simulink model "Exo_Origianl"  (R2023b)
settings: Solver=ode5  StartTime=0.0  StopTime=inf  FixedStep=dt  RelTol=1e-3  EnableMultiTasking=on
values from neighbouring files (symbols this model uses):
  A_0_a = 4.011    [Operator.m]
  A_0_h = 40.69    [Operator.m]
  A_0_k = 25.7    [Operator.m]
  A_1_a = 5.292    [Operator.m]
  A_1_h = 23.22    [Operator.m]
  A_1_k = -3.827    [Operator.m]
  A_2_a = -8.582    [Operator.m]
  A_2_h = -4.487    [Operator.m]
  A_2_k = -8.543    [Operator.m]
  A_3_a = -0.4755    [Operator.m]
  A_3_h = 0.3995    [Operator.m]
  A_3_k = 1.913    [Operator.m]
  A_4_a = 1.688    [Operator.m]
  A_4_k = 1.087    [Operator.m]
  A_5_a = -0.03504    [Operator.m]
  A_5_k = 2.054    [Operator.m]
  A_6_a = 1.298    [Operator.m]
  A_6_k = -0.3061    [Operator.m]
  amplitude = 0.8    [Operator.m]
  ankleStrategyInterval = 1.5    [Operator.m]
  B_1_a = 3.613    [Operator.m]
  B_1_h = -8.65    [Operator.m]
  B_1_k = -19.28    [Operator.m]
  B_2_a = -5.954    [Operator.m]
  B_2_h = 3.338    [Operator.m]
  B_2_k = 17.93    [Operator.m]
  B_3_a = 5.918    [Operator.m]
  B_3_h = 1.389    [Operator.m]
  B_3_k = 3.772    [Operator.m]
  B_4_a = -2.118    [Operator.m]
  B_4_k = 1.504    [Operator.m]
  B_5_a = 1.023    [Operator.m]
  B_5_k = 0.5838    [Operator.m]
  B_6_a = -0.7245    [Operator.m]
  B_6_k = -0.8958    [Operator.m]
  DCM_filter = 1 - dt/(dt+RC)    (= 0.926612305411)    [Operator.m]
  dt = 0.01    [Operator.m]
  frequency = 1.2    [Operator.m]
  gamma = fzero(eqn, 0.1)    [Operator.m]
  hipOffset = -17    [Operator.m]
  K_high = 0.5    [Operator.m]
  K_low = 0.5    [Operator.m]
  KD = 0.39    [Operator.m]
  Kp = 10    [Operator.m]
  l3 = userHeight*0.232    (= 15.776)    [Operator.m]
  l4 = userHeight*0.247    (= 16.796)    [Operator.m]
  l_c2 = ((0.29*34.66+0.63*6.07)/(6.07+34.66))/(0.52+0.19)*l2    (= 15.0425832454)    [Operator.m]
  l_c3 = 0.17/0.40*l3    (= 6.7048)    [Operator.m]
  l_c4 = ((0.19*3.52+0.43*1.05)/(3.52+1.05))/0.43*l4    (= 9.57536959951)    [Operator.m]
  l_foot = 11.25    [Operator.m]
  m2 = m2 + 2.2048*7.591    (= 119.8566368)    [Operator.m]
  m3 = m3 + 2.2048*1.715    (= 19.781232)    [Operator.m]
  m4 = userWeight*(0.0459+0.0169)    (= 10.048)    [Operator.m]
  m_Exo = 2.2048*1.647    (= 3.6313056)    [Operator.m]
  m_f = userWeight*0.0169    (= 2.704)    [Operator.m]
  maxTorque = 35    [Operator.m]
  P_t_ZMP_gain_Ankle = 0    [Operator.m]
  P_t_ZMP_gain_Hip = 0    [Operator.m]
  Phase_Left = 2+pi    (= 5.14159265359)    [Operator.m]
  Phase_Right = 2    [Operator.m]
  ramp = 2    [Operator.m]
  Strategy_filter = DCM_filter    (= 0.926612305411)    [Operator.m]
  strategySaturation = 10    [Operator.m]
  userHeight = 68    [Operator.m]
  userWeight = 160    [Operator.m]
undefined symbols (not defined in the file or in its folder): CAN_Device, DCMErrorPenalty, PEAK, Phase_Left_Knee_0, System, totalPowerPenalty
libraries: sldrtlib x35, simulink x16, rllib x1
(part 3 of 4)

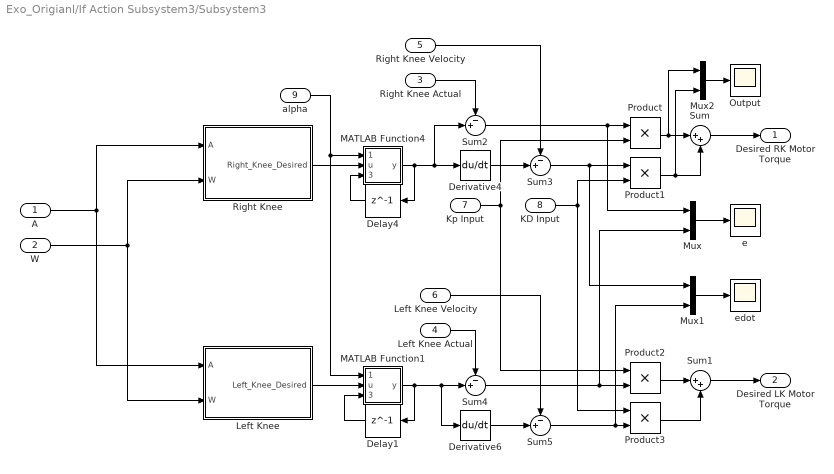
== system Exo_Origianl/If Action Subsystem3/Subsystem3 ==
  A : Inport
  W : Inport  Port=2
  Right Knee Actual : Inport  Port=3
  Left Knee Actual : Inport  Port=4
  Right Knee Velocity : Inport  Port=5
  Left Knee Velocity : Inport  Port=6
  Kp Input : Inport  Port=7
  KD Input : Inport  Port=8
  alpha : Inport  Port=9
  Delay1 : Delay  DelayLength=1
  Delay4 : Delay  DelayLength=1
  Derivative4 : Derivative
  Derivative6 : Derivative
  Left Knee : Subsystem
  MATLAB Function1 : MATLAB Function  TreatAsAtomicUnit=on
  MATLAB Function4 : MATLAB Function  TreatAsAtomicUnit=on
  Mux : Mux  Inputs=2
  Mux1 : Mux  Inputs=2
  Mux2 : Mux  Inputs=2
  Output : Scope
  Product{,1..3} (4 alike) : Product
  Right Knee : Subsystem
  Sum : Sum  Inputs=|++
  Sum1 : Sum  Inputs=|++
  Sum{2..5} (4 alike) : Sum  Inputs=-+|
  e : Scope
  edot : Scope
  Desired RK Motor Torque : Outport
  Desired LK Motor Torque : Outport  Port=2
  wires:
  KD Input/1 -> Product3/1, Product1/2
  Kp Input/1 -> Product2/1, Product/2
  Product3/1 -> Sum1/2
  W/1 -> Left Knee/2(W), Right Knee/2(W)
  Product1/1 -> Mux2/2, Sum/2
  Sum4/1 -> Mux/2, Product2/2
  Sum/1 -> Desired RK Motor Torque/1
  Sum2/1 -> Mux/1, Product/1
  Product/1 -> Mux2/1, Sum/1
  Product2/1 -> Sum1/1
  Sum3/1 -> Mux1/1, Product1/1
  Sum1/1 -> Desired LK Motor Torque/1
  Sum5/1 -> Mux1/2, Product3/2
  Mux/1 -> e/1
  Mux1/1 -> edot/1
  Right Knee Actual/1 -> Sum2/1
  Derivative4/1 -> Sum3/2
  Right Knee Velocity/1 -> Sum3/1
  Left Knee Actual/1 -> Sum4/1
  Derivative6/1 -> Sum5/2
  Left Knee Velocity/1 -> Sum5/1
  Mux2/1 -> Output/1
  MATLAB Function4/1(y) -> Sum2/2, Derivative4/1, Delay4/1
  MATLAB Function1/1(y) -> Derivative6/1, Sum4/2, Delay1/1
  A/1 -> Right Knee/1(A), Left Knee/1(A)
  Right Knee/1(Right_Knee_Desired) -> MATLAB Function4/2(u)
  Delay4/1 -> MATLAB Function4/3(y_delay)
  alpha/1 -> MATLAB Function4/1(alpha), MATLAB Function1/1(alpha)
  Left Knee/1(Left_Knee_Desired) -> MATLAB Function1/2(u)
  Delay1/1 -> MATLAB Function1/3(y_delay)

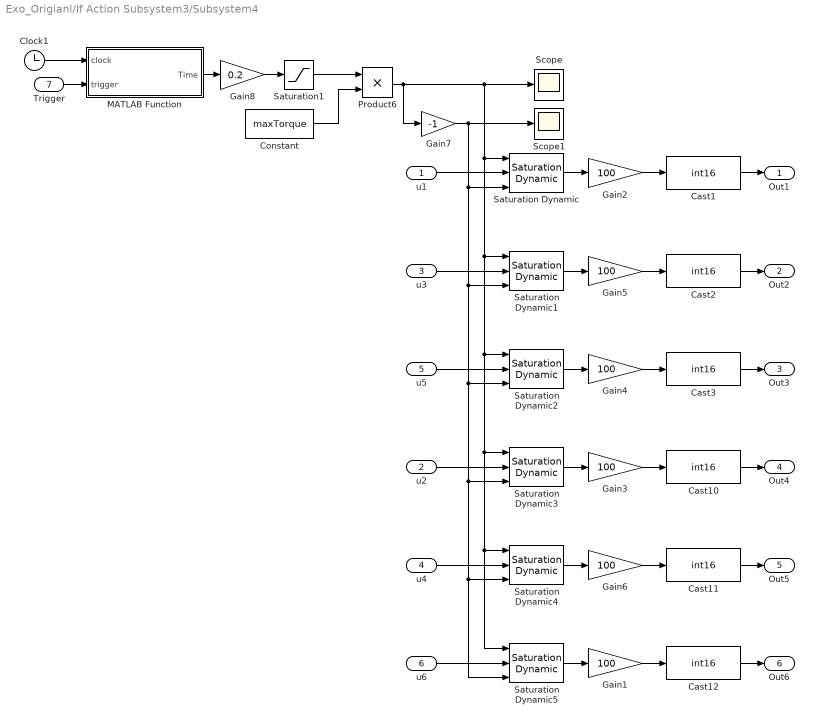
== system Exo_Origianl/If Action Subsystem3/Subsystem4 ==
  u1 : Inport
  u2 : Inport  Port=2
  u3 : Inport  Port=3
  u4 : Inport  Port=4
  u5 : Inport  Port=5
  u6 : Inport  Port=6
  Trigger : Inport  Port=7
  Cast{1..3,10..12} (6 alike) : DataTypeConversion  OutDataTypeStr=int16  SaturateOnIntegerOverflow=off  RndMeth=Floor
  Clock1 : Clock
  Constant : Constant  Value=maxTorque
  Gain{1..6} (6 alike) : Gain  Gain=100
  Gain7 : Gain  Gain=-1
  Gain8 : Gain  Gain=0.2
  MATLAB Function : MATLAB Function  TreatAsAtomicUnit=on
  Product6 : Product
  Saturation Dynamic{,1..5} (6 alike) : simulink/Discontinuities/Saturation Dynamic  OutMin=[]  OutMax=[]  OutDataTypeStr=Inherit: Same as second input  OutDataType=fixdt(1, 16)  OutScaling=2^-10  DoSatur=off
  Saturation1 : Saturate  UpperLimit=1  LowerLimit=0
  Scope : Scope
  Scope1 : Scope
  Out1 : Outport
  Out2 : Outport  Port=2
  Out3 : Outport  Port=3
  Out4 : Outport  Port=4
  Out5 : Outport  Port=5
  Out6 : Outport  Port=6
  wires:
  Gain2/1 -> Cast1/1
  Cast10/1 -> Out4/1
  Cast11/1 -> Out5/1
  Gain4/1 -> Cast3/1
  Gain3/1 -> Cast10/1
  Cast3/1 -> Out3/1
  Cast12/1 -> Out6/1
  Gain5/1 -> Cast2/1
  Gain6/1 -> Cast11/1
  Cast1/1 -> Out1/1
  Gain1/1 -> Cast12/1
  Cast2/1 -> Out2/1
  Saturation Dynamic/1 -> Gain2/1
  Saturation Dynamic1/1 -> Gain5/1
  Saturation Dynamic2/1 -> Gain4/1
  Saturation Dynamic3/1 -> Gain3/1
  Saturation Dynamic4/1 -> Gain6/1
  Saturation Dynamic5/1 -> Gain1/1
  Product6/1 -> Scope/1, Saturation Dynamic5/1, Saturation Dynamic4/1, Saturation Dynamic3/1, Saturation Dynamic2/1, Saturation Dynamic1/1, Saturation Dynamic/1, Gain7/1
  Gain7/1 -> Saturation Dynamic5/3, Saturation Dynamic4/3, Saturation Dynamic3/3, Saturation Dynamic2/3, Saturation Dynamic1/3, Saturation Dynamic/3, Scope1/1
  Gain8/1 -> Saturation1/1
  Clock1/1 -> MATLAB Function/1(clock)
  u1/1 -> Saturation Dynamic/2
  u3/1 -> Saturation Dynamic1/2
  u5/1 -> Saturation Dynamic2/2
  u2/1 -> Saturation Dynamic3/2
  u4/1 -> Saturation Dynamic4/2
  u6/1 -> Saturation Dynamic5/2
  Constant/1 -> Product6/2
  Saturation1/1 -> Product6/1
  MATLAB Function/1(Time) -> Gain8/1
  Trigger/1 -> MATLAB Function/2(trigger)

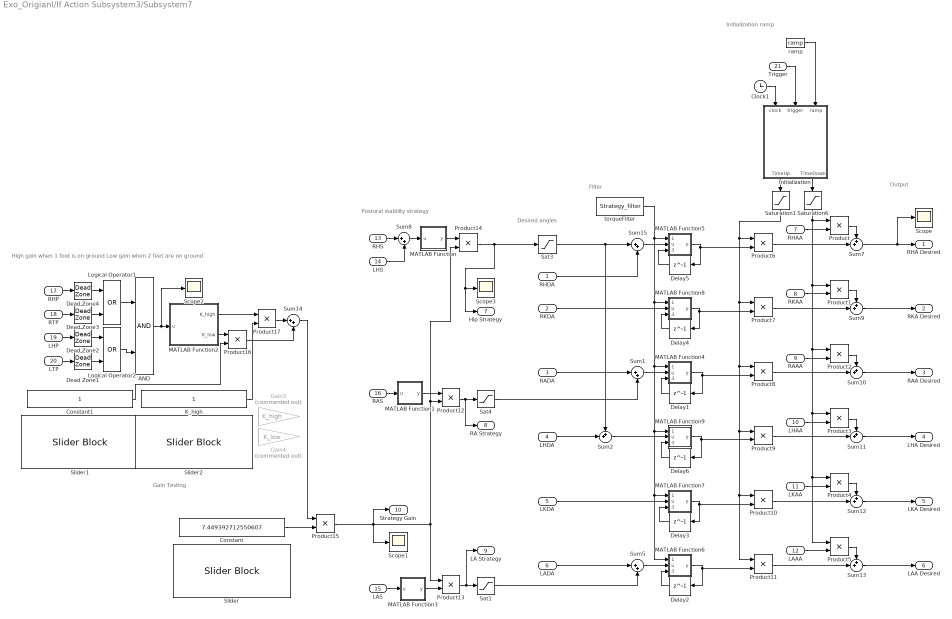
== system Exo_Origianl/If Action Subsystem3/Subsystem7 ==
  note: Gain Testing
  note: Output
  note: Initialization ramp
  note: Filter
  note: Desired angles
  note: Postural stability strategy
  note: High gain when 1 foot is on ground
      | Low gain when 2 feet are on ground
  RHDA : Inport
  RKDA : Inport  Port=2
  RADA : Inport  Port=3
  LHDA : Inport  Port=4
  LKDA : Inport  Port=5
  LADA : Inport  Port=6
  RHAA : Inport  Port=7
  RKAA : Inport  Port=8
  RAAA : Inport  Port=9
  LHAA : Inport  Port=10
  LKAA : Inport  Port=11
  LAAA : Inport  Port=12
  RHS : Inport  Port=13
  LHS : Inport  Port=14
  LAS : Inport  Port=15
  RAS : Inport  Port=16
  RHP : Inport  Port=17
  RTP : Inport  Port=18
  LHP : Inport  Port=19
  LTP : Inport  Port=20
  Trigger : Inport  Port=21
  AND : Logic  IconShape=distinctive  AllPortsSameDT=off  OutDataTypeStr=boolean
  Clock1 : Clock
  Constant : Constant  Value=7.449392712550607
  Constant1 : Constant
  Dead Zone{1..4} (4 alike) : DeadZone  LowerValue=0  UpperValue=pressureDeadZone
  Delay{1..6} (6 alike) : Delay  DelayLength=1
  Gain3 : Gain  Commented=on  Gain=K_high
  Gain4 : Gain  Commented=on  Gain=K_low
  Initialization : MATLAB Function  TreatAsAtomicUnit=on
  K_high : Constant
  Logical Operator1 : Logic  Operator=OR  AllPortsSameDT=off  OutDataTypeStr=boolean
  Logical Operator2 : Logic  Operator=OR  AllPortsSameDT=off  OutDataTypeStr=boolean
  MATLAB Function : MATLAB Function  TreatAsAtomicUnit=on
  MATLAB Function1 : MATLAB Function  TreatAsAtomicUnit=on
  MATLAB Function2 : MATLAB Function  TreatAsAtomicUnit=on
  MATLAB Function3 : MATLAB Function  TreatAsAtomicUnit=on
  MATLAB Function4 : MATLAB Function  TreatAsAtomicUnit=on
  MATLAB Function5 : MATLAB Function  TreatAsAtomicUnit=on
  MATLAB Function6 : MATLAB Function  TreatAsAtomicUnit=on
  MATLAB Function7 : MATLAB Function  TreatAsAtomicUnit=on
  MATLAB Function8 : MATLAB Function  TreatAsAtomicUnit=on
  MATLAB Function9 : MATLAB Function  TreatAsAtomicUnit=on
  Product{,1..17} (18 alike) : Product
  Sat1 : Saturate  UpperLimit=strategySaturation  LowerLimit=-strategySaturation
  Sat3 : Saturate  UpperLimit=strategySaturation  LowerLimit=-strategySaturation
  Sat4 : Saturate  UpperLimit=strategySaturation  LowerLimit=-strategySaturation
  Saturation1 : Saturate  UpperLimit=1  LowerLimit=0
  Saturation6 : Saturate  UpperLimit=1  LowerLimit=0
  Scope{,1..3} (4 alike) : Scope
  Slider : SliderBlock  ScaleMax=10
  Slider1 : SliderBlock  ScaleMin=0.5  ScaleMax=1
  Slider2 : SliderBlock  ScaleMin=1  ScaleMax=3
  Sum{1,5,8,14..15} (5 alike) : Sum  Inputs=|++
  Sum{2,7,9..13} (7 alike) : Sum  Inputs=++|
  ramp : Constant  Value=ramp
  torqueFilter : Constant  Value=Strategy_filter
  RHA Desired : Outport
  RKA Desired : Outport  Port=2
  RAA Desired : Outport  Port=3
  LHA Desired : Outport  Port=4
  LKA Desired : Outport  Port=5
  LAA Desired : Outport  Port=6
  Hip Strategy : Outport  Port=7
  RA Strategy : Outport  Port=8
  LA Strategy : Outport  Port=9
  Strategy Gain : Outport  Port=10
  wires:
  RHS/1 -> Sum8/1
  LADA/1 -> Sum5/1
  LHDA/1 -> Sum2/2
  Sum2/1 -> MATLAB Function9/2(u)
  Sum13/1 -> LAA Desired/1
  Sum8/1 -> MATLAB Function/1(u)
  MATLAB Function6/1(y) -> Product11/2, Delay2/1
  RAS/1 -> MATLAB Function1/1(u)
  MATLAB Function4/1(y) -> Product8/2, Delay1/1
  MATLAB Function1/1(y) -> Product12/1
  Sum11/1 -> LHA Desired/1
  Sum7/1 -> RHA Desired/1, Scope/1
  Sum9/1 -> RKA Desired/1
  Sum10/1 -> RAA Desired/1
  Sum12/1 -> LKA Desired/1
  RADA/1 -> Sum1/1
  LHS/1 -> Sum8/2
  LAS/1 -> MATLAB Function3/1(u)
  RKDA/1 -> MATLAB Function8/2(u)
  LKDA/1 -> MATLAB Function7/2(u)
  Trigger/1 -> Initialization/2(trigger)
  Clock1/1 -> Initialization/1(clock)
  RHAA/1 -> Product/2
  RKAA/1 -> Product1/2
  RAAA/1 -> Product2/2
  LHAA/1 -> Product3/2
  LKAA/1 -> Product4/2
  LAAA/1 -> Product5/2
  Initialization/2(TimeDown) -> Saturation6/1
  Delay5/1 -> MATLAB Function5/3(y_delay)
  torqueFilter/1 -> MATLAB Function5/1(alpha), MATLAB Function9/1(alpha), MATLAB Function7/1(alpha), MATLAB Function6/1(alpha), MATLAB Function4/1(alpha), MATLAB Function8/1(alpha)
  Delay1/1 -> MATLAB Function4/3(y_delay)
  Delay2/1 -> MATLAB Function6/3(y_delay)
  MATLAB Function5/1(y) -> Product6/2, Delay5/1
  RHP/1 -> Dead Zone4/1
  RTP/1 -> Dead Zone3/1
  LHP/1 -> Dead Zone2/1
  LTP/1 -> Dead Zone1/1
  Logical Operator1/1 -> AND/1
  Product12/1 -> Sat4/1, RA Strategy/1
  Product13/1 -> LA Strategy/1, Sat1/1
  Logical Operator2/1 -> AND/2
  MATLAB Function3/1(y) -> Product13/2
  Saturation6/1 -> Product5/1, Product4/1, Product3/1, Product2/1, Product1/1, Product/1
  Product/1 -> Sum7/1
  Product1/1 -> Sum9/1
  Product2/1 -> Sum10/1
  Product3/1 -> Sum11/1
  Product4/1 -> Sum12/1
  Product5/1 -> Sum13/1
  Dead Zone4/1 -> Logical Operator1/1
  Dead Zone3/1 -> Logical Operator1/2
  Dead Zone2/1 -> Logical Operator2/1
  Dead Zone1/1 -> Logical Operator2/2
  MATLAB Function2/1(K_high) -> Product17/1
  MATLAB Function2/2(K_low) -> Product16/1
  Product16/1 -> Sum14/2
  Product17/1 -> Sum14/1
  ramp/1 -> Initialization/3(ramp)
  AND/1 -> Scope2/1, MATLAB Function2/1(u)
  Sum15/1 -> MATLAB Function5/2(u)
  RHDA/1 -> Sum15/2
  Sum5/1 -> MATLAB Function6/2(u)
  Delay3/1 -> MATLAB Function7/3(y_delay)
  MATLAB Function7/1(y) -> Product10/2, Delay3/1
  Sum1/1 -> MATLAB Function4/2(u)
  Delay4/1 -> MATLAB Function8/3(y_delay)
  MATLAB Function8/1(y) -> Product7/2, Delay4/1
  Delay6/1 -> MATLAB Function9/3(y_delay)
  MATLAB Function9/1(y) -> Product9/2, Delay6/1
  Initialization/1(TimeUp) -> Saturation1/1
  Product6/1 -> Sum7/2
  Saturation1/1 -> Product10/1, Product11/1, Product9/1, Product8/1, Product7/1, Product6/1
  Product7/1 -> Sum9/2
  Product8/1 -> Sum10/2
  Product9/1 -> Sum11/2
  Product10/1 -> Sum12/2
  Product11/1 -> Sum13/2
  Product14/1 -> Scope3/1, Hip Strategy/1, Sat3/1
  MATLAB Function/1(y) -> Product14/1
  Product15/1 -> Scope1/1, Strategy Gain/1, Product14/2, Product12/2, Product13/1
  Sat3/1 -> Sum2/1, Sum15/1
  Sat4/1 -> Sum1/2
  Sat1/1 -> Sum5/2
  Sum14/1 -> Product15/1
  Constant/1 -> Product15/2
  Constant1/1 -> Product16/2
  K_high/1 -> Product17/2

== system Exo_Origianl/Read Angular Possition/If Action Subsystem ==
  Action Port : ActionPort  ActionPortLabel=if(u1 == 1)
  Data Type Conversion{6..11} (6 alike) : DataTypeConversion  OutDataTypeStr=double  SaturateOnIntegerOverflow=off  RndMeth=Floor
  Packet Input1 : sldrtlib/Packet Input  SampleTime=-1  MaxMissedTicks=10  ShowMissedTicks=off  YieldWhenWaiting=off  DrvName=PEAK-System/CAN_Device  DrvAddress=81  DrvOptions=[0 0 0 0 1000 0 0 1 5 2 1 3 1]  PacketSize=6  DataTypes={'int8','int8','int8','int8','int8','int8'}  ShowReady=off  ShowError=off  PacketID=2048e0 + (110)  ByteOrder=1  ShowTimestamp=off
      settings: AttributesFormatString=PEAK-System\nCAN Device [81]
  Out7 : Outport
  Out8 : Outport  Port=2
  Out9 : Outport  Port=3
  Out10 : Outport  Port=4
  Out11 : Outport  Port=5
  Out12 : Outport  Port=6
  wires:
  Data Type Conversion10/1 -> Out11/1
  Packet Input1/6 -> Data Type Conversion11/1
  Data Type Conversion11/1 -> Out12/1
  Packet Input1/5 -> Data Type Conversion10/1
  Data Type Conversion7/1 -> Out8/1
  Packet Input1/4 -> Data Type Conversion9/1
  Data Type Conversion6/1 -> Out7/1
  Packet Input1/2 -> Data Type Conversion7/1
  Data Type Conversion8/1 -> Out9/1
  Packet Input1/1 -> Data Type Conversion6/1
  Data Type Conversion9/1 -> Out10/1
  Packet Input1/3 -> Data Type Conversion8/1

== system Exo_Origianl/Read Angular Possition/If Action Subsystem1 ==
  Action Port : ActionPort  ActionPortLabel=else
  Data Type Conversion{6..11} (6 alike) : DataTypeConversion  OutDataTypeStr=double  SaturateOnIntegerOverflow=off  RndMeth=Floor
  Multiply{,1..5} (6 alike) : Gain  Gain=0.1
  Packet Input1 : sldrtlib/Packet Input  SampleTime=-1  MaxMissedTicks=10000  ShowMissedTicks=off  YieldWhenWaiting=off  DrvName=PEAK-System/CAN_Device  DrvAddress=81  DrvOptions=[0 0 0 0 1000 0 0 1 5 2 1 3 1]  PacketSize=6  DataTypes={'int16','int16','int16'}  ShowReady=off  ShowError=off  PacketID=2048e0 + (50)  ByteOrder=1  ShowTimestamp=off
      settings: AttributesFormatString=PEAK-System\nCAN Device [81]
  Packet Input2 : sldrtlib/Packet Input  SampleTime=-1  MaxMissedTicks=1000  ShowMissedTicks=off  YieldWhenWaiting=off  DrvName=PEAK-System/CAN_Device  DrvAddress=81  DrvOptions=[0 0 0 0 1000 0 0 1 5 2 1 3 1]  PacketSize=6  DataTypes={'int16','int16','int16'}  ShowReady=off  ShowError=off  PacketID=2048e0 + (51)  ByteOrder=1  ShowTimestamp=off
      settings: AttributesFormatString=PEAK-System\nCAN Device [81]
  Out7 : Outport
  Out8 : Outport  Port=2
  Out9 : Outport  Port=3
  Out10 : Outport  Port=4
  Out11 : Outport  Port=5
  Out12 : Outport  Port=6
  wires:
  Packet Input2/1 -> Data Type Conversion9/1
  Packet Input1/3 -> Data Type Conversion8/1
  Packet Input1/2 -> Data Type Conversion7/1
  Packet Input2/3 -> Data Type Conversion11/1
  Packet Input2/2 -> Data Type Conversion10/1
  Packet Input1/1 -> Data Type Conversion6/1
  Data Type Conversion6/1 -> Multiply/1
  Multiply/1 -> Out7/1
  Data Type Conversion7/1 -> Multiply1/1
  Multiply1/1 -> Out8/1
  Data Type Conversion8/1 -> Multiply2/1
  Multiply2/1 -> Out9/1
  Data Type Conversion9/1 -> Multiply3/1
  Multiply3/1 -> Out10/1
  Data Type Conversion10/1 -> Multiply4/1
  Multiply4/1 -> Out11/1
  Data Type Conversion11/1 -> Multiply5/1
  Multiply5/1 -> Out12/1

== system Exo_Origianl/Read Angular Velocity/If Action Subsystem1 ==
  Action Port : ActionPort  ActionPortLabel=else
  Data Type Conversion{6..11} (6 alike) : DataTypeConversion  OutDataTypeStr=double  SaturateOnIntegerOverflow=off  RndMeth=Floor
  Multiply{,1..5} (6 alike) : Gain  Gain=0.1
  Packet Input1 : sldrtlib/Packet Input  SampleTime=-1  MaxMissedTicks=10000  ShowMissedTicks=off  YieldWhenWaiting=off  DrvName=PEAK-System/CAN_Device  DrvAddress=81  DrvOptions=[0 0 0 0 1000 0 0 1 5 2 1 3 1]  PacketSize=6  DataTypes={'int16','int16','int16'}  ShowReady=off  ShowError=off  PacketID=2048e0 + (52)  ByteOrder=1  ShowTimestamp=off
      settings: AttributesFormatString=PEAK-System\nCAN Device [81]
  Packet Input2 : sldrtlib/Packet Input  SampleTime=-1  MaxMissedTicks=1000  ShowMissedTicks=off  YieldWhenWaiting=off  DrvName=PEAK-System/CAN_Device  DrvAddress=81  DrvOptions=[0 0 0 0 1000 0 0 1 5 2 1 3 1]  PacketSize=6  DataTypes={'int16','int16','int16'}  ShowReady=off  ShowError=off  PacketID=2048e0 + (53)  ByteOrder=1  ShowTimestamp=off
      settings: AttributesFormatString=PEAK-System\nCAN Device [81]
  Out7 : Outport
  Out8 : Outport  Port=2
  Out9 : Outport  Port=3
  Out10 : Outport  Port=4
  Out11 : Outport  Port=5
  Out12 : Outport  Port=6
  wires:
  Packet Input2/1 -> Data Type Conversion9/1
  Packet Input1/3 -> Data Type Conversion8/1
  Packet Input1/2 -> Data Type Conversion7/1
  Packet Input2/3 -> Data Type Conversion11/1
  Packet Input2/2 -> Data Type Conversion10/1
  Packet Input1/1 -> Data Type Conversion6/1
  Data Type Conversion6/1 -> Multiply/1
  Multiply/1 -> Out7/1
  Data Type Conversion7/1 -> Multiply1/1
  Multiply1/1 -> Out8/1
  Data Type Conversion8/1 -> Multiply2/1
  Multiply2/1 -> Out9/1
  Data Type Conversion9/1 -> Multiply3/1
  Multiply3/1 -> Out10/1
  Data Type Conversion10/1 -> Multiply4/1
  Multiply4/1 -> Out11/1
  Data Type Conversion11/1 -> Multiply5/1
  Multiply5/1 -> Out12/1

== system Exo_Origianl/Read Interaction torque/If Action Subsystem ==
  Action Port : ActionPort  ActionPortLabel=if(u1 == 1)
  Data Type Conversion{6..11} (6 alike) : DataTypeConversion  OutDataTypeStr=double  SaturateOnIntegerOverflow=off  RndMeth=Floor
  Packet Input1 : sldrtlib/Packet Input  SampleTime=-1  MaxMissedTicks=10  ShowMissedTicks=off  YieldWhenWaiting=off  DrvName=PEAK-System/CAN_Device  DrvAddress=81  DrvOptions=[0 0 0 0 1000 0 0 1 5 2 1 3 1]  PacketSize=6  DataTypes={'int8','int8','int8','int8','int8','int8'}  ShowReady=off  ShowError=off  PacketID=2048e0 + (120)  ByteOrder=1  ShowTimestamp=off
      settings: AttributesFormatString=PEAK-System\nCAN Device [81]
  Out7 : Outport
  Out8 : Outport  Port=2
  Out9 : Outport  Port=3
  Out10 : Outport  Port=4
  Out11 : Outport  Port=5
  Out12 : Outport  Port=6
  wires:
  Data Type Conversion10/1 -> Out11/1
  Packet Input1/6 -> Data Type Conversion11/1
  Data Type Conversion11/1 -> Out12/1
  Packet Input1/5 -> Data Type Conversion10/1
  Data Type Conversion7/1 -> Out8/1
  Packet Input1/4 -> Data Type Conversion9/1
  Data Type Conversion6/1 -> Out7/1
  Packet Input1/2 -> Data Type Conversion7/1
  Data Type Conversion8/1 -> Out9/1
  Packet Input1/1 -> Data Type Conversion6/1
  Data Type Conversion9/1 -> Out10/1
  Packet Input1/3 -> Data Type Conversion8/1

== system Exo_Origianl/Read Interaction torque/If Action Subsystem1 ==
  Action Port : ActionPort  ActionPortLabel=else
  Data Type Conversion{6..11} (6 alike) : DataTypeConversion  OutDataTypeStr=double  SaturateOnIntegerOverflow=off  RndMeth=Floor
  Multiply{,1..5} (6 alike) : Gain  Gain=0.1
  Packet Input1 : sldrtlib/Packet Input  SampleTime=-1  MaxMissedTicks=10000  ShowMissedTicks=off  YieldWhenWaiting=off  DrvName=PEAK-System/CAN_Device  DrvAddress=81  DrvOptions=[0 0 0 0 1000 0 0 1 5 2 1 3 1]  PacketSize=6  DataTypes={'int16','int16','int16'}  ShowReady=off  ShowError=off  PacketID=2048e0 + (54)  ByteOrder=1  ShowTimestamp=off
      settings: AttributesFormatString=PEAK-System\nCAN Device [81]
  Packet Input2 : sldrtlib/Packet Input  SampleTime=-1  MaxMissedTicks=1000  ShowMissedTicks=off  YieldWhenWaiting=off  DrvName=PEAK-System/CAN_Device  DrvAddress=81  DrvOptions=[0 0 0 0 1000 0 0 1 5 2 1 3 1]  PacketSize=6  DataTypes={'int16','int16','int16'}  ShowReady=off  ShowError=off  PacketID=2048e0 + (55)  ByteOrder=1  ShowTimestamp=off
      settings: AttributesFormatString=PEAK-System\nCAN Device [81]
  Out7 : Outport
  Out8 : Outport  Port=2
  Out9 : Outport  Port=3
  Out10 : Outport  Port=4
  Out11 : Outport  Port=5
  Out12 : Outport  Port=6
  wires:
  Packet Input2/1 -> Data Type Conversion9/1
  Packet Input1/3 -> Data Type Conversion8/1
  Packet Input1/2 -> Data Type Conversion7/1
  Packet Input2/3 -> Data Type Conversion11/1
  Packet Input2/2 -> Data Type Conversion10/1
  Packet Input1/1 -> Data Type Conversion6/1
  Data Type Conversion6/1 -> Multiply/1
  Multiply/1 -> Out7/1
  Data Type Conversion7/1 -> Multiply1/1
  Multiply1/1 -> Out8/1
  Data Type Conversion8/1 -> Multiply2/1
  Multiply2/1 -> Out9/1
  Data Type Conversion9/1 -> Multiply3/1
  Multiply3/1 -> Out10/1
  Data Type Conversion10/1 -> Multiply4/1
  Multiply4/1 -> Out11/1
  Data Type Conversion11/1 -> Multiply5/1
  Multiply5/1 -> Out12/1

== system Exo_Origianl/Read Motor torque/If Action Subsystem ==
  Action Port : ActionPort  ActionPortLabel=if(u1 == 1)
  Data Type Conversion{6..11} (6 alike) : DataTypeConversion  OutDataTypeStr=double  SaturateOnIntegerOverflow=off  RndMeth=Floor
  Packet Input1 : sldrtlib/Packet Input  SampleTime=-1  MaxMissedTicks=10  ShowMissedTicks=off  YieldWhenWaiting=off  DrvName=PEAK-System/CAN_Device  DrvAddress=81  DrvOptions=[0 0 0 0 1000 0 0 1 5 2 1 3 1]  PacketSize=6  DataTypes={'int8','int8','int8','int8','int8','int8'}  ShowReady=off  ShowError=off  PacketID=2048e0 + (140)  ByteOrder=1  ShowTimestamp=off
      settings: AttributesFormatString=PEAK-System\nCAN Device [81]
  Out7 : Outport
  Out8 : Outport  Port=2
  Out9 : Outport  Port=3
  Out10 : Outport  Port=4
  Out11 : Outport  Port=5
  Out12 : Outport  Port=6
  wires:
  Data Type Conversion10/1 -> Out11/1
  Packet Input1/6 -> Data Type Conversion11/1
  Data Type Conversion11/1 -> Out12/1
  Packet Input1/5 -> Data Type Conversion10/1
  Data Type Conversion7/1 -> Out8/1
  Packet Input1/4 -> Data Type Conversion9/1
  Data Type Conversion6/1 -> Out7/1
  Packet Input1/2 -> Data Type Conversion7/1
  Data Type Conversion8/1 -> Out9/1
  Packet Input1/1 -> Data Type Conversion6/1
  Data Type Conversion9/1 -> Out10/1
  Packet Input1/3 -> Data Type Conversion8/1

== system Exo_Origianl/Read Motor torque/If Action Subsystem1 ==
  Action Port : ActionPort  ActionPortLabel=else
  Data Type Conversion{6..11} (6 alike) : DataTypeConversion  OutDataTypeStr=double  SaturateOnIntegerOverflow=off  RndMeth=Floor
  Multiply{,1..5} (6 alike) : Gain  Gain=0.1
  Packet Input1 : sldrtlib/Packet Input  SampleTime=-1  MaxMissedTicks=10000  ShowMissedTicks=off  YieldWhenWaiting=off  DrvName=PEAK-System/CAN_Device  DrvAddress=81  DrvOptions=[0 0 0 0 1000 0 0 1 5 2 1 3 1]  PacketSize=6  DataTypes={'int16','int16','int16'}  ShowReady=off  ShowError=off  PacketID=2048e0 + (56)  ByteOrder=1  ShowTimestamp=off
      settings: AttributesFormatString=PEAK-System\nCAN Device [81]
  Packet Input2 : sldrtlib/Packet Input  SampleTime=-1  MaxMissedTicks=1000  ShowMissedTicks=off  YieldWhenWaiting=off  DrvName=PEAK-System/CAN_Device  DrvAddress=81  DrvOptions=[0 0 0 0 1000 0 0 1 5 2 1 3 1]  PacketSize=6  DataTypes={'int16','int16','int16'}  ShowReady=off  ShowError=off  PacketID=2048e0 + (57)  ByteOrder=1  ShowTimestamp=off
      settings: AttributesFormatString=PEAK-System\nCAN Device [81]
  Out7 : Outport
  Out8 : Outport  Port=2
  Out9 : Outport  Port=3
  Out10 : Outport  Port=4
  Out11 : Outport  Port=5
  Out12 : Outport  Port=6
  wires:
  Packet Input2/1 -> Data Type Conversion9/1
  Packet Input1/3 -> Data Type Conversion8/1
  Packet Input1/2 -> Data Type Conversion7/1
  Packet Input2/3 -> Data Type Conversion11/1
  Packet Input2/2 -> Data Type Conversion10/1
  Packet Input1/1 -> Data Type Conversion6/1
  Data Type Conversion6/1 -> Multiply/1
  Multiply/1 -> Out7/1
  Data Type Conversion7/1 -> Multiply1/1
  Multiply1/1 -> Out8/1
  Data Type Conversion8/1 -> Multiply2/1
  Multiply2/1 -> Out9/1
  Data Type Conversion9/1 -> Multiply3/1
  Multiply3/1 -> Out10/1
  Data Type Conversion10/1 -> Multiply4/1
  Multiply4/1 -> Out11/1
  Data Type Conversion11/1 -> Multiply5/1
  Multiply5/1 -> Out12/1

== system Exo_Origianl/Subsystem13/Subsystem14 ==
  DCM Error : Inport
  Power : Inport  Port=2
  "                    " : Gain  Gain=-totalPowerPenalty
  "                    1" : Gain  Gain=-DCMErrorPenalty
  Bus Creator1 : BusCreator  Inputs=2
  Constant : Constant  Value=4
  Constant1 : Constant  Value=2
  Math Function : Math  Operator=pow
  Math Function2 : Math  Operator=pow
  Sum of Elements : Sum  Inputs=+
  Reward : Outport  VectorParamsAs1DForOutWhenUnconnected=off
  wires:
  Power/1 -> Math Function2/2
  Constant1/1 -> Math Function2/1
  Constant/1 -> Math Function/1
  DCM Error/1 -> Math Function/2
  Math Function2/1 -> "                    "/1
  Math Function/1 -> "                    1"/1
  Sum of Elements/1 -> Reward/1
  Bus Creator1/1 -> Sum of Elements/1
  "                    1"/1 -> Bus Creator1/1  "DCM Penalty"
  "                    "/1 -> Bus Creator1/2  "Power Penalty"

== system Exo_Origianl/Subsystem15/Subsystem14 ==
  Input : Inport
  Constant12 : Constant  Value=0
  Constant3 : Constant
  Display4 : Display
  If Action Subsystem4 : Subsystem  TreatAsAtomicUnit=on
  If Action Subsystem5 : Subsystem  TreatAsAtomicUnit=on
  If Action Subsystem6 : Subsystem  TreatAsAtomicUnit=on
  If Action Subsystem7 : Subsystem  TreatAsAtomicUnit=on
  If Action Subsystem8 : Subsystem  TreatAsAtomicUnit=on
  If3 : If  IfExpression=u1 == 0  ElseIfExpressions=u1 == 11, u1 == 12, u1 == 19
  Merge1 : Merge  Inputs=5
  Out1 : Outport
  wires:
  Constant12/1 -> If Action Subsystem8/1(In1)
  If Action Subsystem4/1(Out1) -> Merge1/1
  If3/3 -> If Action Subsystem6/Action
  If3/4 -> If Action Subsystem7/Action
  If Action Subsystem5/1(Out1) -> Merge1/2
  If Action Subsystem7/1(Out1) -> Merge1/4
  If3/5 -> If Action Subsystem8/Action
  If3/1 -> If Action Subsystem4/Action
  Input/1 -> If3/1
  Merge1/1 -> Out1/1, Display4/1
  If Action Subsystem8/1(Out1) -> Merge1/5
  If3/2 -> If Action Subsystem5/Action
  Constant3/1 -> If Action Subsystem7/1(In1), If Action Subsystem6/1(In1), If Action Subsystem5/1(In1), If Action Subsystem4/1(In1)
  If Action Subsystem6/1(Out1) -> Merge1/3

== system Exo_Origianl/Up and Down Assistance % Left/Subsystem ==
  In1 : Inport
  In2 : Inport  Port=2
  Add : Sum  OutMin=[0]  OutMax=[10]
  Add1 : Sum  OutMin=[0]  OutMax=[10]
  Add2 : Sum
  Cast To Double : DataTypeConversion  OutDataTypeStr=double  SaturateOnIntegerOverflow=off  RndMeth=Floor
  Constant : Constant  Value=10
  Constant1 : Constant  Value=40
  Delay : Delay  DelayLength=1
  Delay1 : Delay  DelayLength=1
  Detect Rise Positive : simulink/Logic and Bit Operations/Detect Rise Positive  vinit=0  OutDataTypeStr=uint8
  Detect Rise Positive1 : simulink/Logic and Bit Operations/Detect Rise Positive  vinit=0  OutDataTypeStr=uint8
  Display1 : Display
  Display2 : Display
  Gain : Gain  Gain=10
  If : If  IfExpression=(u1 > 0)
  If Action Subsystem : Subsystem  TreatAsAtomicUnit=on
  If Action Subsystem1 : Subsystem  TreatAsAtomicUnit=on
  If1 : If  IfExpression=(u1 < 9)
  Minus : Sum  Inputs=+-
  Minus1 : Sum  Inputs=+-  OutMin=[0]  OutMax=[10]
  Out1 : Outport
  Out2 : Outport  Port=2
  wires:
  Detect Rise Positive1/1 -> Minus1/2
  Detect Rise Positive/1 -> Add/2
  Minus1/1 -> Delay1/1
  Add/1 -> Delay/1
  Add1/1 -> Cast To Double/1
  Cast To Double/1 -> If/1, Minus/2, If1/1, Display2/1
  If Action Subsystem/1(Out1) -> Detect Rise Positive/1
  If1/1 -> If Action Subsystem/Action
  If Action Subsystem1/1(Out1) -> Detect Rise Positive1/1
  If/1 -> If Action Subsystem1/Action
  In1/1 -> If Action Subsystem/1(In1)
  In2/1 -> If Action Subsystem1/1(In1)
  Delay/1 -> Add1/1, Display1/1, Add/1
  Delay1/1 -> Minus1/1, Add1/2
  Gain/1 -> Out1/1
  Constant/1 -> Minus/1
  Minus/1 -> Add2/1, Gain/1
  Constant1/1 -> Add2/2
  Add2/1 -> Out2/1

== system Exo_Origianl/Up and Down Assistance % Right/Subsystem ==
  In1 : Inport
  In2 : Inport  Port=2
  Add : Sum  OutMin=[0]  OutMax=[10]
  Add1 : Sum  OutMin=[0]  OutMax=[10]
  Add2 : Sum
  Cast To Double : DataTypeConversion  OutDataTypeStr=double  SaturateOnIntegerOverflow=off  RndMeth=Floor
  Constant : Constant  Value=10
  Constant1 : Constant  Value=30
  Delay : Delay  DelayLength=1
  Delay1 : Delay  DelayLength=1
  Detect Rise Positive : simulink/Logic and Bit Operations/Detect Rise Positive  vinit=0  OutDataTypeStr=uint8
  Detect Rise Positive1 : simulink/Logic and Bit Operations/Detect Rise Positive  vinit=0  OutDataTypeStr=uint8
  Display1 : Display
  Display2 : Display
  Gain : Gain  Gain=10
  If : If  IfExpression=(u1 > 0)
  If Action Subsystem : Subsystem  TreatAsAtomicUnit=on
  If Action Subsystem1 : Subsystem  TreatAsAtomicUnit=on
  If1 : If  IfExpression=(u1 < 9)
  Minus : Sum  Inputs=+-
  Minus1 : Sum  Inputs=+-  OutMin=[0]  OutMax=[10]
  Out1 : Outport
  Out2 : Outport  Port=2
  wires:
  Detect Rise Positive1/1 -> Minus1/2
  Detect Rise Positive/1 -> Add/2
  Minus1/1 -> Delay1/1
  Add/1 -> Delay/1
  Add1/1 -> Cast To Double/1
  Cast To Double/1 -> If/1, Minus/2, If1/1, Display2/1
  If Action Subsystem/1(Out1) -> Detect Rise Positive/1
  If1/1 -> If Action Subsystem/Action
  If Action Subsystem1/1(Out1) -> Detect Rise Positive1/1
  If/1 -> If Action Subsystem1/Action
  In1/1 -> If Action Subsystem/1(In1)
  In2/1 -> If Action Subsystem1/1(In1)
  Delay/1 -> Add1/1, Display1/1, Add/1
  Delay1/1 -> Minus1/1, Add1/2
  Gain/1 -> Out1/1
  Constant/1 -> Minus/1
  Minus/1 -> Add2/1, Gain/1
  Add2/1 -> Out2/1
  Constant1/1 -> Add2/2

== system Exo_Origianl/Up and Down Speed/Subsystem ==
  In1 : Inport
  In2 : Inport  Port=2
  Add : Sum  OutMin=[0]  OutMax=[10]
  Add1 : Sum  OutMin=[0]  OutMax=[10]
  Cast To Double : DataTypeConversion  OutDataTypeStr=double  SaturateOnIntegerOverflow=off  RndMeth=Floor
  Delay : Delay  DelayLength=1
  Delay1 : Delay  DelayLength=1
  Detect Rise Positive : simulink/Logic and Bit Operations/Detect Rise Positive  vinit=0  OutDataTypeStr=uint8
  Detect Rise Positive1 : simulink/Logic and Bit Operations/Detect Rise Positive  vinit=0  OutDataTypeStr=uint8
  Display1 : Display
  Display2 : Display
  If : If  IfExpression=(u1 > 1)
  If Action Subsystem : Subsystem  TreatAsAtomicUnit=on
  If Action Subsystem1 : Subsystem  TreatAsAtomicUnit=on
  If1 : If  IfExpression=(u1 < 10)
  Increment Stored Integer : simulink/Additional Math & Discrete/Additional Math: Increment - Decrement/Increment Stored Integer
  Minus1 : Sum  Inputs=+-  OutMin=[0]  OutMax=[10]
  Out1 : Outport
  wires:
  Detect Rise Positive1/1 -> Minus1/2
  Detect Rise Positive/1 -> Add/2
  Minus1/1 -> Delay1/1
  Delay/1 -> Add1/1, Display1/1, Add/1
  Add/1 -> Delay/1
  Delay1/1 -> Add1/2, Minus1/1
  Add1/1 -> Increment Stored Integer/1
  Increment Stored Integer/1 -> Cast To Double/1
  Cast To Double/1 -> If/1, Out1/1, If1/1, Display2/1
  If Action Subsystem/1(Out1) -> Detect Rise Positive/1
  If1/1 -> If Action Subsystem/Action
  If Action Subsystem1/1(Out1) -> Detect Rise Positive1/1
  If/1 -> If Action Subsystem1/Action
  In1/1 -> If Action Subsystem/1(In1)
  In2/1 -> If Action Subsystem1/1(In1)

== system Exo_Origianl/If Action Subsystem3/Fourier Series/Left Ankle ==
  A : Inport
  W : Inport  Port=2
  Constant : Constant  Value=Phase_Left
  Integrator1 : Integrator  ExternalReset=rising  InitialConditionSource=external  InitialCondition=Phase_Left_Knee_0
  Mux1 : Mux  Inputs=2
  Scope1 : Scope
  ankle walk : Fcn  Expr=u(1)*(A_0_a + A_1_a*cos(u(2)) + B_1_a*sin(u(2)) + A_2_a*cos(2*u(2)) + B_2_a*sin(2*u(2)) + A_3_a*cos(3*u(2)) + B_3_a*sin(3*u(2)) + A_4_a*cos(4*u(2)) + B_4_a*sin(4*u(2)) + A_5_a*cos(5*u(2)) + B_5_a*sin(5*u(2)) + A_6_a*cos(6*u(2)) + B_6_a*sin(6*u(2)))
  Left_Ankle_Desired : Outport
  wires:
  W/1 -> Integrator1/2, Integrator1/1
  Mux1/1 -> ankle walk/1
  Constant/1 -> Integrator1/3
  A/1 -> Mux1/1
  ankle walk/1 -> Left_Ankle_Desired/1
  Integrator1/1 -> Mux1/2, Scope1/1

== system Exo_Origianl/If Action Subsystem3/Fourier Series/Left Hip ==
  A : Inport
  W : Inport  Port=2
  Offset : Inport  Port=3
  Constant1 : Constant  Value=Phase_Left
  Integrator4 : Integrator  ExternalReset=rising  InitialConditionSource=external  InitialCondition=Phase_Left_Knee_0
  Mux6 : Mux  Inputs=3
  Scope : Scope
  hip walk : Fcn  Expr=(u(1)*(A_0_h + A_1_h*cos(u(2)) + A_2_h*cos(2*u(2)) + A_3_h*cos(3*u(2)) + B_1_h*sin(u(2)) + B_2_h*sin(2*u(2)) + B_3_h*sin(3*u(2))))+u(3)
  Left_Hip_Desired : Outport
  wires:
  W/1 -> Integrator4/2, Integrator4/1
  Mux6/1 -> hip walk/1
  Constant1/1 -> Integrator4/3
  A/1 -> Mux6/1
  hip walk/1 -> Left_Hip_Desired/1
  Offset/1 -> Mux6/3
  Integrator4/1 -> Scope/1, Mux6/2

== system Exo_Origianl/If Action Subsystem3/Fourier Series/Left Knee ==
  A : Inport
  W : Inport  Port=2
  Constant1 : Constant  Value=Phase_Left
  Integrator1 : Integrator  ExternalReset=rising  InitialConditionSource=external  InitialCondition=Phase_Left_Knee_0
  Mux1 : Mux  Inputs=2
  Scope4 : Scope
  knee walk : Fcn  Expr=u(1)*(A_0_k + A_1_k*cos(u(2)) + B_1_k*sin(u(2)) + A_2_k*cos(2*u(2)) + B_2_k*sin(2*u(2)) + A_3_k*cos(3*u(2)) + B_3_k*sin(3*u(2)) + A_4_k*cos(4*u(2)) + B_4_k*sin(4*u(2)) + A_5_k*cos(5*u(2)) + B_5_k*sin(5*u(2)) + A_6_k*cos(6*u(2)) + B_6_k*sin(6*u(2)))
  Left_Knee_Desired : Outport
  wires:
  A/1 -> Mux1/1
  W/1 -> Integrator1/2, Integrator1/1
  Integrator1/1 -> Mux1/2, Scope4/1
  Constant1/1 -> Integrator1/3
  Mux1/1 -> knee walk/1
  knee walk/1 -> Left_Knee_Desired/1

== system Exo_Origianl/If Action Subsystem3/Fourier Series/Right Ankle ==
  A : Inport
  W : Inport  Port=2
  Constant : Constant  Value=Phase_Right
  Integrator1 : Integrator  ExternalReset=rising  InitialConditionSource=external  InitialCondition=Phase_Left_Knee_0
  Mux1 : Mux  Inputs=2
  Scope1 : Scope
  ankle walk : Fcn  Expr=u(1)*(A_0_a + A_1_a*cos(u(2)) + B_1_a*sin(u(2)) + A_2_a*cos(2*u(2)) + B_2_a*sin(2*u(2)) + A_3_a*cos(3*u(2)) + B_3_a*sin(3*u(2)) + A_4_a*cos(4*u(2)) + B_4_a*sin(4*u(2)) + A_5_a*cos(5*u(2)) + B_5_a*sin(5*u(2)) + A_6_a*cos(6*u(2)) + B_6_a*sin(6*u(2)))
  Right_Ankle_Desired : Outport
  wires:
  W/1 -> Integrator1/2, Integrator1/1
  Mux1/1 -> ankle walk/1
  Constant/1 -> Integrator1/3
  A/1 -> Mux1/1
  ankle walk/1 -> Right_Ankle_Desired/1
  Integrator1/1 -> Mux1/2, Scope1/1

== system Exo_Origianl/If Action Subsystem3/Fourier Series/Right Hip ==
  A : Inport
  W : Inport  Port=2
  Offset : Inport  Port=3
  Constant1 : Constant  Value=Phase_Right
  Integrator4 : Integrator  ExternalReset=rising  InitialConditionSource=external  InitialCondition=Phase_Left_Knee_0
  Mux6 : Mux  Inputs=3
  Scope : Scope
  hip walk : Fcn  Expr=(u(1)*(A_0_h + A_1_h*cos(u(2)) + A_2_h*cos(2*u(2)) + A_3_h*cos(3*u(2)) + B_1_h*sin(u(2)) + B_2_h*sin(2*u(2)) + B_3_h*sin(3*u(2))))+u(3)
  Right_Hip_Desired : Outport
  wires:
  W/1 -> Integrator4/2, Integrator4/1
  Mux6/1 -> hip walk/1
  Constant1/1 -> Integrator4/3
  A/1 -> Mux6/1
  hip walk/1 -> Right_Hip_Desired/1
  Offset/1 -> Mux6/3
  Integrator4/1 -> Scope/1, Mux6/2

== system Exo_Origianl/If Action Subsystem3/Fourier Series/Right Knee ==
  W : Inport
  A : Inport  Port=2
  Constant1 : Constant  Value=Phase_Right
  Integrator1 : Integrator  ExternalReset=rising  InitialConditionSource=external  InitialCondition=Phase_Left_Knee_0
  Mux1 : Mux  Inputs=2
  Scope4 : Scope
  knee walk : Fcn  Expr=u(1)*(A_0_k + A_1_k*cos(u(2)) + B_1_k*sin(u(2)) + A_2_k*cos(2*u(2)) + B_2_k*sin(2*u(2)) + A_3_k*cos(3*u(2)) + B_3_k*sin(3*u(2)) + A_4_k*cos(4*u(2)) + B_4_k*sin(4*u(2)) + A_5_k*cos(5*u(2)) + B_5_k*sin(5*u(2)) + A_6_k*cos(6*u(2)) + B_6_k*sin(6*u(2)))
  Right_Knee_Desired : Outport
  wires:
  A/1 -> Mux1/1
  W/1 -> Integrator1/2, Integrator1/1
  Constant1/1 -> Integrator1/3
  Mux1/1 -> knee walk/1
  knee walk/1 -> Right_Knee_Desired/1
  Integrator1/1 -> Mux1/2, Scope4/1

== system Exo_Origianl/If Action Subsystem3/Subsystem/Left Ankle ==
  A : Inport
  W : Inport  Port=2
  Constant : Constant  Value=Phase_Left
  Integrator1 : Integrator  ExternalReset=rising  InitialConditionSource=external  InitialCondition=Phase_Left_Knee_0
  Mux1 : Mux  Inputs=2
  Scope1 : Scope
  ankle walk : Fcn  Expr=u(1)*(A_0_a + A_1_a*cos(u(2)) + B_1_a*sin(u(2)) + A_2_a*cos(2*u(2)) + B_2_a*sin(2*u(2)) + A_3_a*cos(3*u(2)) + B_3_a*sin(3*u(2)) + A_4_a*cos(4*u(2)) + B_4_a*sin(4*u(2)) + A_5_a*cos(5*u(2)) + B_5_a*sin(5*u(2)) + A_6_a*cos(6*u(2)) + B_6_a*sin(6*u(2)))
  Left_Ankle_Desired : Outport
  wires:
  W/1 -> Integrator1/2, Integrator1/1
  Mux1/1 -> ankle walk/1
  Constant/1 -> Integrator1/3
  A/1 -> Mux1/1
  ankle walk/1 -> Left_Ankle_Desired/1
  Integrator1/1 -> Mux1/2, Scope1/1

== system Exo_Origianl/If Action Subsystem3/Subsystem/Right Ankle ==
  A : Inport
  W : Inport  Port=2
  Constant : Constant  Value=Phase_Right
  Integrator1 : Integrator  ExternalReset=rising  InitialConditionSource=external  InitialCondition=Phase_Left_Knee_0
  Mux1 : Mux  Inputs=2
  Scope1 : Scope
  ankle walk : Fcn  Expr=u(1)*(A_0_a + A_1_a*cos(u(2)) + B_1_a*sin(u(2)) + A_2_a*cos(2*u(2)) + B_2_a*sin(2*u(2)) + A_3_a*cos(3*u(2)) + B_3_a*sin(3*u(2)) + A_4_a*cos(4*u(2)) + B_4_a*sin(4*u(2)) + A_5_a*cos(5*u(2)) + B_5_a*sin(5*u(2)) + A_6_a*cos(6*u(2)) + B_6_a*sin(6*u(2)))
  Right_Ankle_Desired : Outport
  wires:
  W/1 -> Integrator1/2, Integrator1/1
  Mux1/1 -> ankle walk/1
  Constant/1 -> Integrator1/3
  A/1 -> Mux1/1
  ankle walk/1 -> Right_Ankle_Desired/1
  Integrator1/1 -> Mux1/2, Scope1/1

== system Exo_Origianl/If Action Subsystem3/Subsystem1/Left Hip ==
  A : Inport
  W : Inport  Port=2
  Offset : Inport  Port=3
  Constant1 : Constant  Value=Phase_Left
  Integrator4 : Integrator  ExternalReset=rising  InitialConditionSource=external  InitialCondition=Phase_Left_Knee_0
  Mux6 : Mux  Inputs=3
  Scope : Scope
  hip walk : Fcn  Expr=(u(1)*(A_0_h + A_1_h*cos(u(2)) + A_2_h*cos(2*u(2)) + A_3_h*cos(3*u(2)) + B_1_h*sin(u(2)) + B_2_h*sin(2*u(2)) + B_3_h*sin(3*u(2))))+u(3)
  Left_Hip_Desired : Outport
  wires:
  W/1 -> Integrator4/2, Integrator4/1
  Mux6/1 -> hip walk/1
  Constant1/1 -> Integrator4/3
  A/1 -> Mux6/1
  hip walk/1 -> Left_Hip_Desired/1
  Offset/1 -> Mux6/3
  Integrator4/1 -> Scope/1, Mux6/2

== system Exo_Origianl/If Action Subsystem3/Subsystem1/Right Hip ==
  A : Inport
  W : Inport  Port=2
  Offset : Inport  Port=3
  Constant1 : Constant  Value=Phase_Right
  Integrator4 : Integrator  ExternalReset=rising  InitialConditionSource=external  InitialCondition=Phase_Left_Knee_0
  Mux6 : Mux  Inputs=3
  Scope : Scope
  hip walk : Fcn  Expr=(u(1)*(A_0_h + A_1_h*cos(u(2)) + A_2_h*cos(2*u(2)) + A_3_h*cos(3*u(2)) + B_1_h*sin(u(2)) + B_2_h*sin(2*u(2)) + B_3_h*sin(3*u(2))))+u(3)
  Right_Hip_Desired : Outport
  wires:
  W/1 -> Integrator4/2, Integrator4/1
  Mux6/1 -> hip walk/1
  Constant1/1 -> Integrator4/3
  A/1 -> Mux6/1
  hip walk/1 -> Right_Hip_Desired/1
  Offset/1 -> Mux6/3
  Integrator4/1 -> Scope/1, Mux6/2

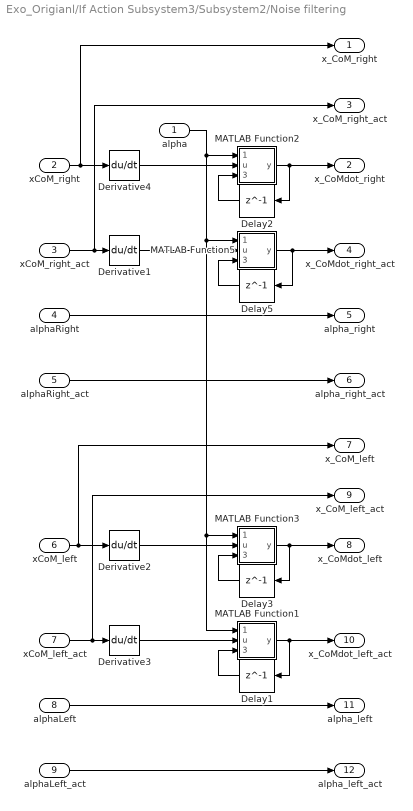
== system Exo_Origianl/If Action Subsystem3/Subsystem2/Noise filtering ==
  alpha : Inport
  xCoM_right : Inport  Port=2
  xCoM_right_act : Inport  Port=3
  alphaRight : Inport  Port=4
  alphaRight_act : Inport  Port=5
  xCoM_left : Inport  Port=6
  xCoM_left_act : Inport  Port=7
  alphaLeft : Inport  Port=8
  alphaLeft_act : Inport  Port=9
  Delay{1..3,5} (4 alike) : Delay  DelayLength=1
  Derivative{1..4} (4 alike) : Derivative
  MATLAB Function1 : MATLAB Function  TreatAsAtomicUnit=on
  MATLAB Function2 : MATLAB Function  TreatAsAtomicUnit=on
  MATLAB Function3 : MATLAB Function  TreatAsAtomicUnit=on
  MATLAB Function5 : MATLAB Function  TreatAsAtomicUnit=on
  x_CoM_right : Outport
  x_CoMdot_right : Outport  Port=2
  x_CoM_right_act : Outport  Port=3
  x_CoMdot_right_act : Outport  Port=4
  alpha_right : Outport  Port=5
  alpha_right_act : Outport  Port=6
  x_CoM_left : Outport  Port=7
  x_CoMdot_left : Outport  Port=8
  x_CoM_left_act : Outport  Port=9
  x_CoMdot_left_act : Outport  Port=10
  alpha_left : Outport  Port=11
  alpha_left_act : Outport  Port=12
  wires:
  Derivative1/1 -> MATLAB Function5/2(u)
  Derivative2/1 -> MATLAB Function3/2(u)
  Derivative4/1 -> MATLAB Function2/2(u)
  Delay5/1 -> MATLAB Function5/3(y_delay)
  alpha/1 -> MATLAB Function2/1(alpha), MATLAB Function3/1(alpha), MATLAB Function1/1(alpha), MATLAB Function5/1(alpha)
  xCoM_right_act/1 -> x_CoM_right_act/1, Derivative1/1
  xCoM_right/1 -> Derivative4/1, x_CoM_right/1
  xCoM_left_act/1 -> x_CoM_left_act/1, Derivative3/1
  xCoM_left/1 -> x_CoM_left/1, Derivative2/1
  Delay1/1 -> MATLAB Function1/3(y_delay)
  Derivative3/1 -> MATLAB Function1/2(u)
  alphaRight/1 -> alpha_right/1
  alphaRight_act/1 -> alpha_right_act/1
  alphaLeft_act/1 -> alpha_left_act/1
  alphaLeft/1 -> alpha_left/1
  MATLAB Function1/1(y) -> x_CoMdot_left_act/1, Delay1/1
  MATLAB Function5/1(y) -> Delay5/1, x_CoMdot_right_act/1
  MATLAB Function2/1(y) -> x_CoMdot_right/1, Delay2/1
  Delay2/1 -> MATLAB Function2/3(y_delay)
  MATLAB Function3/1(y) -> Delay3/1, x_CoMdot_left/1
  Delay3/1 -> MATLAB Function3/3(y_delay)

== system Exo_Origianl/If Action Subsystem3/Subsystem2/Subsystem6 ==
  x_CoM_right : Inport
  x_CoM_right_act : Inport  Port=2
  xdot_CoM_right : Inport  Port=3
  xdot_CoM_right_act : Inport  Port=4
  alpha_right : Inport  Port=5
  alpha_right_act : Inport  Port=6
  zeta_t_err_Right : Inport  Port=7
  CoM Right : Inport  Port=8
  x_CoM_left : Inport  Port=9
  x_CoM_left_act : Inport  Port=10
  xdot_CoM_left : Inport  Port=11
  xdot_CoM_left_act : Inport  Port=12
  alpha_left : Inport  Port=13
  alpha_left_act : Inport  Port=14
  zeta_t_err_Left : Inport  Port=15
  CoM Left : Inport  Port=16
  DCM : Inport  Port=17
  DCM_act : Inport  Port=18
  Mux2 : Mux  Inputs=18
  Out1 : Outport
  wires:
  x_CoM_left_act/1 -> Mux2/10
  CoM Right/1 -> Mux2/8
  x_CoM_left/1 -> Mux2/9
  Mux2/1 -> Out1/1
  alpha_left/1 -> Mux2/13
  alpha_left_act/1 -> Mux2/14
  x_CoM_right/1 -> Mux2/1
  zeta_t_err_Left/1 -> Mux2/15
  xdot_CoM_left/1 -> Mux2/11
  DCM/1 -> Mux2/17
  CoM Left/1 -> Mux2/16
  alpha_right/1 -> Mux2/5
  alpha_right_act/1 -> Mux2/6
  zeta_t_err_Right/1 -> Mux2/7
  xdot_CoM_right/1 -> Mux2/3
  x_CoM_right_act/1 -> Mux2/2
  xdot_CoM_left_act/1 -> Mux2/12
  xdot_CoM_right_act/1 -> Mux2/4
  DCM_act/1 -> Mux2/18

== system Exo_Origianl/If Action Subsystem3/Subsystem3/Left Knee ==
  A : Inport
  W : Inport  Port=2
  Constant1 : Constant  Value=Phase_Left
  Integrator1 : Integrator  ExternalReset=rising  InitialConditionSource=external  InitialCondition=Phase_Left_Knee_0
  Mux1 : Mux  Inputs=2
  Scope4 : Scope
  knee walk : Fcn  Expr=u(1)*(A_0_k + A_1_k*cos(u(2)) + B_1_k*sin(u(2)) + A_2_k*cos(2*u(2)) + B_2_k*sin(2*u(2)) + A_3_k*cos(3*u(2)) + B_3_k*sin(3*u(2)) + A_4_k*cos(4*u(2)) + B_4_k*sin(4*u(2)) + A_5_k*cos(5*u(2)) + B_5_k*sin(5*u(2)) + A_6_k*cos(6*u(2)) + B_6_k*sin(6*u(2)))
  Left_Knee_Desired : Outport
  wires:
  knee walk/1 -> Left_Knee_Desired/1
  W/1 -> Integrator1/2, Integrator1/1
  Mux1/1 -> knee walk/1
  A/1 -> Mux1/1
  Constant1/1 -> Integrator1/3
  Integrator1/1 -> Mux1/2, Scope4/1

== system Exo_Origianl/If Action Subsystem3/Subsystem3/Right Knee ==
  A : Inport
  W : Inport  Port=2
  Constant2 : Constant  Value=Phase_Right
  Integrator1 : Integrator  ExternalReset=rising  InitialConditionSource=external  InitialCondition=Phase_Left_Knee_0
  Mux1 : Mux  Inputs=2
  Scope4 : Scope
  knee walk : Fcn  Expr=u(1)*(A_0_k + A_1_k*cos(u(2)) + B_1_k*sin(u(2)) + A_2_k*cos(2*u(2)) + B_2_k*sin(2*u(2)) + A_3_k*cos(3*u(2)) + B_3_k*sin(3*u(2)) + A_4_k*cos(4*u(2)) + B_4_k*sin(4*u(2)) + A_5_k*cos(5*u(2)) + B_5_k*sin(5*u(2)) + A_6_k*cos(6*u(2)) + B_6_k*sin(6*u(2)))
  Right_Knee_Desired : Outport
  wires:
  knee walk/1 -> Right_Knee_Desired/1
  Constant2/1 -> Integrator1/3
  A/1 -> Mux1/1
  W/1 -> Integrator1/2, Integrator1/1
  Integrator1/1 -> Mux1/2, Scope4/1
  Mux1/1 -> knee walk/1

== system Exo_Origianl/Subsystem15/Subsystem14/If Action Subsystem4 ==
  In1 : Inport
  Action Port : ActionPort  ActionPortLabel=if(u1 == 0)
  Out1 : Outport
  wires:
  In1/1 -> Out1/1

== system Exo_Origianl/Subsystem15/Subsystem14/If Action Subsystem5 ==
  In1 : Inport
  Action Port : ActionPort  ActionPortLabel=elseif(u1 == 11)
  Out1 : Outport
  wires:
  In1/1 -> Out1/1

== system Exo_Origianl/Subsystem15/Subsystem14/If Action Subsystem6 ==
  In1 : Inport
  Action Port : ActionPort  ActionPortLabel=elseif( u1 == 12)
  Out1 : Outport
  wires:
  In1/1 -> Out1/1

== system Exo_Origianl/Subsystem15/Subsystem14/If Action Subsystem7 ==
  In1 : Inport
  Action Port : ActionPort  ActionPortLabel=elseif( u1 == 19)
  Out1 : Outport
  wires:
  In1/1 -> Out1/1

== system Exo_Origianl/Subsystem15/Subsystem14/If Action Subsystem8 ==
  In1 : Inport
  Action Port : ActionPort  ActionPortLabel=else
  Out1 : Outport
  wires:
  In1/1 -> Out1/1

== system Exo_Origianl/Up and Down Assistance % Left/Subsystem/If Action Subsystem ==
  In1 : Inport
  Action Port : ActionPort  ActionPortLabel=if((u1 < 9))
  Out1 : Outport
  wires:
  In1/1 -> Out1/1

== system Exo_Origianl/Up and Down Assistance % Left/Subsystem/If Action Subsystem1 ==
  In1 : Inport
  Action Port : ActionPort  ActionPortLabel=if((u1 > 0))
  Out1 : Outport
  wires:
  In1/1 -> Out1/1

== system Exo_Origianl/Up and Down Assistance % Right/Subsystem/If Action Subsystem ==
  In1 : Inport
  Action Port : ActionPort  ActionPortLabel=if((u1 < 9))
  Out1 : Outport
  wires:
  In1/1 -> Out1/1

== system Exo_Origianl/Up and Down Assistance % Right/Subsystem/If Action Subsystem1 ==
  In1 : Inport
  Action Port : ActionPort  ActionPortLabel=if((u1 > 0))
  Out1 : Outport
  wires:
  In1/1 -> Out1/1

== system Exo_Origianl/Up and Down Speed/Subsystem/If Action Subsystem ==
  In1 : Inport
  Action Port : ActionPort  ActionPortLabel=if((u1 < 10))
  Out1 : Outport
  wires:
  In1/1 -> Out1/1

== system Exo_Origianl/Up and Down Speed/Subsystem/If Action Subsystem1 ==
  In1 : Inport
  Action Port : ActionPort  ActionPortLabel=if((u1 > 1))
  Out1 : Outport
  wires:
  In1/1 -> Out1/1

== matlab function Exo_Origianl/Subsystem12/MATLAB Function ==
  settings: updateMethod=DISCRETE
  data: clock input; Time output; trigger input
function Time = resetTimer(clock, trigger)
    persistent lastTriggerTime prevTrigger;
    if isempty(lastTriggerTime)
        lastTriggerTime = 0;
    end
    if isempty(prevTrigger)
        prevTrigger = trigger; % Initialize prevTrigger with the current trigger value
    end

    % Reset time when the trigger changes state (either from 0 to 1 or from 1 to 0)
    if trigger ~= prevTrigger
        lastTriggerTime = clock;
    end

    % Update the previous trigger state
    prevTrigger = trigger;

    % Calculate the adjusted time
    Time = clock - lastTriggerTime;
end

== matlab function Exo_Origianl/Subsystem12/MATLAB Function1 ==
  data: clock input; trigger input; amplitude output; ramp input; frequency output; hipOffset output
function [amplitude, frequency, hipOffset] = ramp(clock, trigger, ramp)
    R = 1/ramp;
    if trigger == 1
        amplitude = R*clock;
        frequency = R*clock;
        hipOffset = R*clock;
    else
        amplitude = 1 - R*clock;
        frequency = 1 - R*clock;
        hipOffset = 1 - R*clock;
    end
end

== matlab function Exo_Origianl/If Action Subsystem3/Subsystem1/MATLAB Function2 ==
  data: alpha input; u input; y_delay input; y output
function y = fcn(alpha, u, y_delay)
y = alpha*y_delay + (1-alpha)*u;

== matlab function Exo_Origianl/If Action Subsystem3/Subsystem3/MATLAB Function4 ==
  data: alpha input; u input; y_delay input; y output
function y = fcn(alpha, u, y_delay)
y = alpha*y_delay + (1-alpha)*u;

== matlab function Exo_Origianl/If Action Subsystem3/Subsystem2/Noise filtering/MATLAB Function5 ==
  data: alpha input; u input; y_delay input; y output
function y = fcn(alpha, u, y_delay)
y = alpha*y_delay + (1-alpha)*u;

== matlab function Exo_Origianl/If Action Subsystem3/Subsystem2/Noise filtering/MATLAB Function1 ==
  data: alpha input; u input; y_delay input; y output
function y = fcn(alpha, u, y_delay)
y = alpha*y_delay + (1-alpha)*u;

== matlab function Exo_Origianl/If Action Subsystem3/Subsystem/MATLAB Function3 ==
  data: alpha input; u input; y_delay input; y output
function y = fcn(alpha, u, y_delay)
y = alpha*y_delay + (1-alpha)*u;

== matlab function Exo_Origianl/If Action Subsystem3/Subsystem3/MATLAB Function1 ==
  data: alpha input; u input; y_delay input; y output
function y = fcn(alpha, u, y_delay)
y = alpha*y_delay + (1-alpha)*u;

== matlab function Exo_Origianl/If Action Subsystem3/Subsystem4/MATLAB Function ==
  settings: updateMethod=DISCRETE
  data: clock input; Time output; trigger input
function Time = resetTimer(clock, trigger)
    persistent lastTriggerTime prevTrigger;
    if isempty(lastTriggerTime)
        lastTriggerTime = 0;
    end
    if isempty(prevTrigger)
        prevTrigger = 0;
    end

    if trigger == 1 && prevTrigger ~= 1
        lastTriggerTime = clock;
    end

    prevTrigger = trigger;

    Time = clock - lastTriggerTime;
end
